simulink model "secOrdSS_checkout"  (Simulink 9.2)
settings: Solver=FixedStepDiscrete  StartTime=0.0  StopTime=10  FixedStep=SIM_dt  RelTol=1e-3
values from neighbouring files (symbols this model uses):
  A = sysSS.A    [init_secOrdSS_checkout.m]
  B = sysSS.B    [init_secOrdSS_checkout.m]
  C = sysSS.C    [init_secOrdSS_checkout.m]
  D = sysSS.D    [init_secOrdSS_checkout.m]
  den = [1,2*zeta*w0,w0^2]    [init_secOrdFilt_checkout.m]    (also in init_secOrdSS_checkout.m = sysTF.Denominator)
  num = [0,0,w0^2]    [init_secOrdFilt_checkout.m]    (also in init_secOrdSS_checkout.m = sysTF.Numerator)
  SIM_dt = 0.01    [init_secOrdFilt_checkout.m]    (also in init_secOrdSS_checkout.m = 0.001)
settings Model: Creator=coewal  LastModifiedBy=coewal
settings DataIOCC: LimitDataPoints=off  SaveFormat=Dataset  SignalLoggingSaveFormat=Dataset
settings OptimizationCC: LifeSpan=auto
settings DebuggingCC: UnderspecifiedInitializationDetection=Simplified  MergeDetectMultiDrivingBlocksExec=error  FcnCallInpInsideContextMsg=error  StateNameClashWarn=none  SFUnexpectedBacktrackingDiag=error  SFNoUnconditionalDefaultTransitionDiag=error  SFExecutionAtInitializationDiag=warning
settings HardwareCC: ProdBitPerPointer=64  ProdBitPerSizeT=64  ProdBitPerPtrDiffT=64  ProdLargestAtomicFloat=Float  ProdIntDivRoundTo=Zero  ProdEndianess=LittleEndian  ProdWordSize=64  ProdHWDeviceType=Intel->x86-64 (Windows64)
settings ModelReferenceCC: PropagateSignalLabelsOutOfModel=on
settings SFSimCC: SimUseLocalCustomCode=on
settings RTWCC: RTWUseLocalCustomCode=on
settings CodeAppCC: StateflowObjectComments=off
settings GRTTargetCC: TargetLangStandard=C99 (ISO)  GeneratePreprocessorConditionals=Use local settings  CombineOutputUpdateFcns=on  GRTInterface=off
settings ConfigComp: CovMetricSettings=dwe  CovHtmlReporting=off  CovSaveCumulativeToWorkspaceVar=off  CovSaveSingleToWorkspaceVar=off  CovExternalEMLEnable=on

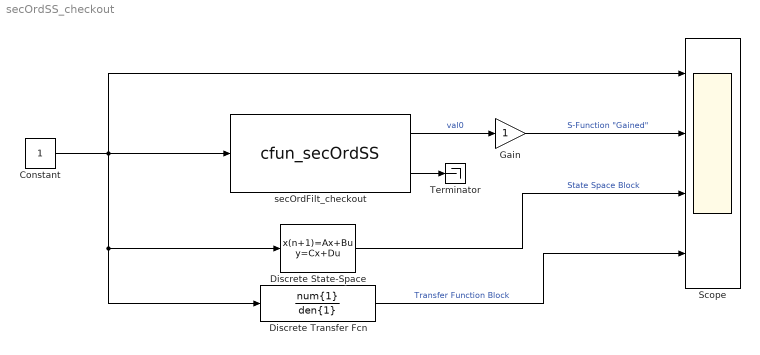
== system secOrdSS_checkout ==
  Constant : Constant
  Discrete Transfer Fcn : DiscreteTransferFcn  Numerator=num{1}  Denominator=den{1}
  Discrete State-Space : DiscreteStateSpace  A=A  B=B  C=C  D=D  SampleTime=SIM_dt
  Gain : Gain
  Scope : Scope  NumInputPorts=4
  Terminator : Terminator
  secOrdFilt_checkout : S-Function  FunctionName=cfun_secOrdSS  Parameters=SIM_dt, A00, A01, A10, A11, B00, B10, C00, C01, C10, C11, D00, D10  SFunctionDeploymentMode=off  EnableBusSupport=off
  wires:
  Constant/1 -> Discrete State-Space/1, Discrete Transfer Fcn/1, Scope/1, secOrdFilt_checkout/1
  secOrdFilt_checkout/1 -> Gain/1  "val0"
  Gain/1 -> Scope/2  "S-Function \"Gained\""
  Discrete State-Space/1 -> Scope/3  "State Space Block"
  Discrete Transfer Fcn/1 -> Scope/4  "Transfer Function Block"
  secOrdFilt_checkout/2 -> Terminator/1
